simulink model "Tp7_ej5_simscape"  (R2023a)
settings: Solver=VariableStepAuto  StartTime=0.0  StopTime=2  RelTol=1e-3
libraries: fl_lib x10, nesl_utility x6, ee_lib x1, SignalEditorBlockLib x1
settings Model: Creator=Juan  LastModifiedBy=Juan

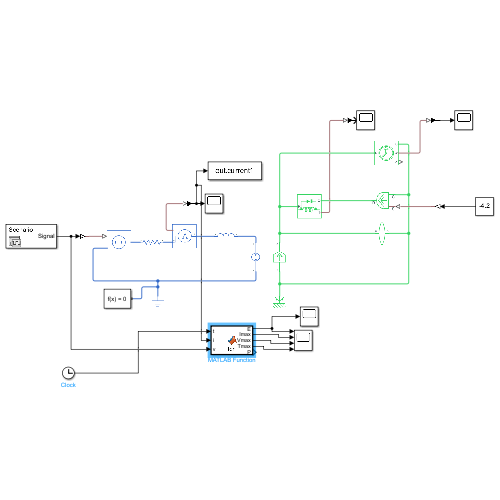
[thumbnail: Simulink's stored preview of the top-level diagram]
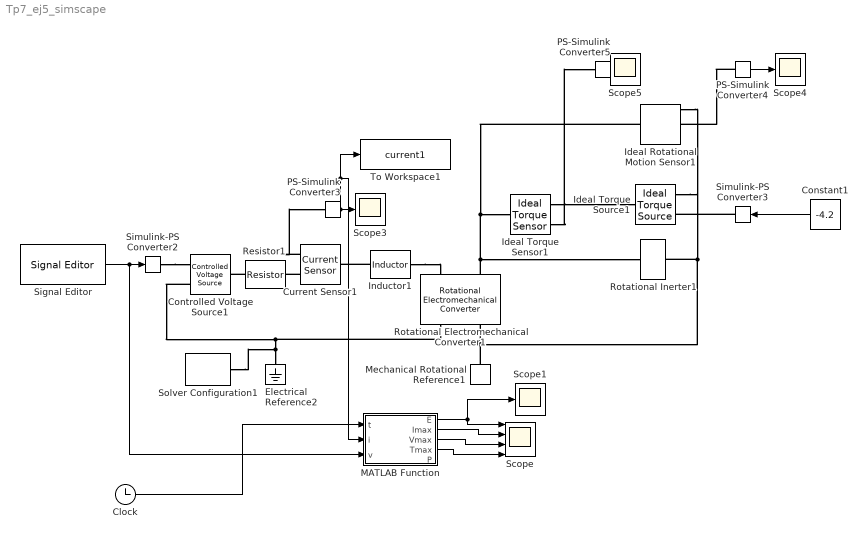
== system Tp7_ej5_simscape ==
  Clock : Clock
  Constant1 : Constant  Value=-4.2
  Controlled Voltage Source1 : fl_lib/Electrical/Electrical Sources/Controlled Voltage Source
  Current Sensor1 : fl_lib/Electrical/Electrical Sensors/Current Sensor
  Electrical Reference2 : fl_lib/Electrical/Electrical Elements/Electrical Reference
  Ideal Rotational Motion Sensor1 : fl_lib/Mechanical/Mechanical Sensors/Ideal Rotational Motion Sensor  reference=foundation.enum.MeasurementReference.difference  acceleration_port=false  velocity_port=true  position_port=true  wrap_angle=false  offset=0 rad
  Ideal Torque Sensor1 : fl_lib/Mechanical/Mechanical Sensors/Ideal Torque Sensor
  Ideal Torque Source1 : fl_lib/Mechanical/Mechanical Sources/Ideal Torque Source
  Inductor1 : ee_lib/Passive/Inductor  l=3 mH  enable_L_tol=ee.enum.toleranceApplication.none  L_tol=20  tol_distribution=ee.enum.toleranceDistribution.uniform  nSigma=4  r=0 Ohm  g=1e-9 1/Ohm  enable_operating_limits=ee.enum.enable.no  operating_limit_action=ee.enum.passive.reportOpLim.warn  max_working_current=1 A  power_rating=1 W  enable_faults=ee.enum.enable.no  fault_action=simscape.enum.assert.action.none  lambdaPercent=50  k_faulted=0.9999  turnsShort=ee.enum.passive.inductor.turnsShortOption.no  openCct=ee.enum.enable.no  groundShort=ee.enum.passive.inductor.groundShortOption.no  groundShortG=0 1/Ohm  tau_fault=1e-3 s  fault_trigger=ee.enum.faults.faultTrigger.temporal  t_fault=1 s  max_permissible_voltage=100 V  n_fail_on_voltage=1  max_permissible_current=1 A  t_fail_on_current=1 s  i_L_specify=off  i_L_priority=High  i_L=0 A  i_L_nominal_specify=off  i_L_nominal_unit=A  i_L_nominal_value=1
  MATLAB Function : MATLAB Function  TreatAsAtomicUnit=on
  Mechanical Rotational Reference1 : fl_lib/Mechanical/Rotational Elements/Mechanical Rotational Reference
  PS-Simulink Converter3 : nesl_utility/PS-Simulink Converter  PhysicalDomain=network_engine_domain  SubClassName=ps_output  LeftPortType=input  RightPortType=output  PseudoPeriodic=off  Frequencies=[]  VectorFormat=inherit  Unit=inherit  AffineConversion=off
  PS-Simulink Converter4 : nesl_utility/PS-Simulink Converter  PhysicalDomain=network_engine_domain  SubClassName=ps_output  LeftPortType=input  RightPortType=output  PseudoPeriodic=off  Frequencies=[]  VectorFormat=inherit  Unit=inherit  AffineConversion=off
  PS-Simulink Converter5 : nesl_utility/PS-Simulink Converter  PhysicalDomain=network_engine_domain  SubClassName=ps_output  LeftPortType=input  RightPortType=output  PseudoPeriodic=off  Frequencies=[]  VectorFormat=inherit  Unit=inherit  AffineConversion=off
  Resistor1 : fl_lib/Electrical/Electrical Elements/Resistor  R=4 Ohm  i_specify=off  i_priority=None  i=0 A  i_nominal_specify=off  i_nominal_unit=A  i_nominal_value=1  v_specify=off  v_priority=None  v=0 V  v_nominal_specify=off  v_nominal_unit=V  v_nominal_value=1
  Rotational Electromechanical Converter1 : fl_lib/Electrical/Electrical Elements/Rotational Electromechanical Converter  K=0.3 V*s/rad  i_specify=off  i_priority=None  i=0 A  i_nominal_specify=off  i_nominal_unit=A  i_nominal_value=1  v_specify=off  v_priority=None  v=0 V  v_nominal_specify=off  v_nominal_unit=V  v_nominal_value=1  t_specify=off  t_priority=None  t=0 N*m  t_nominal_specify=off  t_nominal_unit=N*m  t_nominal_value=1  w_specify=off  w_priority=None  w=0 rad/s  w_nominal_specify=off  w_nominal_unit=rad/s  w_nominal_value=1
  Rotational Inerter1 : fl_lib/Mechanical/Rotational Elements/Rotational Inerter  B=0.215 kg*m^2  w_specify=off  w_priority=High  w=0 rad/s  w_nominal_specify=off  w_nominal_unit=rad/s  w_nominal_value=1  t_specify=off  t_priority=None  t=0 N*m  t_nominal_specify=off  t_nominal_unit=N*m  t_nominal_value=1
      settings: InternalSimscapePortConfiguration="{\"Bottom\":[],\"Left\":[{\"id\":\"R\",\"label\":\"R\",\"type\":\"foundation.mechanical.rotational.rotational\"}],\"Right\":[{\"id\":\"C\",\"label\":\"C\",\"type\":\"foundation.mechanical.rotational.rotational\"}],\"Top\":[]}"
  Scope : Scope  NumInputPorts=4
  Scope{1,3..5} (4 alike) : Scope
  Signal Editor : SignalEditorBlockLib/Signal Editor  FileName=D:\01. Facultad\Control y Sistemas1\Control y Sistemas\Tp7\ej5.mat  ActiveScenario=Scenario  ActiveSignal=Signal  IsBus=off  OutputBusObjectStr=Bus: BusObject  SampleTime=0  Interpolate=off  ZeroCross=off  OutputAfterFinalValue=Setting to zero  Unit=inherit  PreserveSignalName=on  ApplySigPropsToAllScenarios=on
  Simulink-PS Converter2 : nesl_utility/Simulink-PS Converter  PhysicalDomain=network_engine_domain  SubClassName=ps_input  LeftPortType=input  RightPortType=output  PseudoPeriodic=off  Frequencies=[]  NoiseDistribution=none  NoiseParameters=[]  Unit=V  AffineConversion=off  FilteringAndDerivatives=provide  SimscapeFilterOrder=1  InputFilterTimeConstant=0.001  UdotUserProvided=0
  Simulink-PS Converter3 : nesl_utility/Simulink-PS Converter  PhysicalDomain=network_engine_domain  SubClassName=ps_input  LeftPortType=input  RightPortType=output  PseudoPeriodic=off  Frequencies=[]  NoiseDistribution=none  NoiseParameters=[]  Unit=N*m  AffineConversion=off  FilteringAndDerivatives=provide  SimscapeFilterOrder=1  InputFilterTimeConstant=0.001  UdotUserProvided=0
  Solver Configuration1 : nesl_utility/Solver Configuration  PhysicalDomain=network_engine_domain  SubClassName=solver  LeftPortType=input  RightPortType=generic  Tones=[]  Harmonics=[]  SimulateNoise=off  Profile=off  UseLocalSampling=off  EnableSwitchedLinearOptims=on  FrequencyDomain=off  UseCCode=off  RelTol=0.001  AbsTol=0.001  MinStep=1e-09  ToWorkspace=off  RevertToSquareIcSolve=off  NumHomotopyIterations=100  PhasorMode=off  PhasorModeNumHarmonics=1  ConsistencySolver=NEWTON_XTOL_AFTER_FTOL  IndexReductionMethod=DerivativeReplacement  DoDC=off  ResidualTolerance=1e-09  ConsistencyTolSource=GLOBAL  ConsistencyAbsTol=0.001  ConsistencyRelTol=0.001  ConsistencyTolFactor=0.001  UseLocalSolver=off  LocalSolverChoice=NE_BACKWARD_EULER_ADVANCER  ResolveIndetEquations=on  FunctionEvalNumThread=1  LocalSolverSampleTime=0.001  DoFixedCost=off  MaxNonlinIter=3  MaxModeIter=2  ComputeImpulses=off  ImpulseIterations=2  LinearAlgebra=auto  LinearAlgebraNumThread=0  EquationFormulation=NE_TIME_EF  DelaysMemoryBudget=1024  AutomaticFiltering=on  FilteringTimeConstant=0.001  PartitionStorageMethod=AS_NEEDED  PartitionMemoryBudget=1024  PartitionMethod=ROBUST
  To Workspace1 : ToWorkspace  VariableName=current1  SaveFormat=Timeseries  SampleTime=-1
  wires:
  Signal Editor/1 -> MATLAB Function/3(v), Simulink-PS Converter2/1
  PS-Simulink Converter3/1 -> MATLAB Function/2(i), To Workspace1/1, Scope3/1
  Constant1/1 -> Simulink-PS Converter3/1
  PS-Simulink Converter4/1 -> Scope4/1
  Clock/1 -> MATLAB Function/1(t)
  MATLAB Function/1(E) -> Scope/1, Scope1/1
  MATLAB Function/2(Imax) -> Scope/2
  MATLAB Function/3(Vmax) -> Scope/3
  MATLAB Function/4(Tmax) -> Scope/4
  connections:
  Controlled Voltage Source1/RConn2 -- Solver Configuration1/RConn1 -- Electrical Reference2/LConn1 -- Rotational Electromechanical Converter1/RConn1
  Simulink-PS Converter2/RConn1 -- Controlled Voltage Source1/RConn1
  Resistor1/LConn1 -- Controlled Voltage Source1/LConn1
  Inductor1/RConn1 -- Rotational Electromechanical Converter1/LConn1
  Current Sensor1/RConn2 -- Resistor1/RConn1
  Inductor1/LConn1 -- Current Sensor1/LConn1
  Current Sensor1/RConn1 -- PS-Simulink Converter3/LConn1
  Rotational Electromechanical Converter1/LConn2 -- Ideal Torque Sensor1/LConn1 -- Ideal Rotational Motion Sensor1/LConn1 -- Rotational Inerter1/LConn1
  Mechanical Rotational Reference1/LConn1 -- Rotational Electromechanical Converter1/RConn2 -- Ideal Torque Source1/RConn2 -- Ideal Rotational Motion Sensor1/RConn1 -- Rotational Inerter1/RConn1
  Simulink-PS Converter3/RConn1 -- Ideal Torque Source1/RConn1
  Ideal Torque Sensor1/RConn1 -- Ideal Torque Source1/LConn1
  PS-Simulink Converter4/LConn1 -- Ideal Rotational Motion Sensor1/RConn2
  Ideal Torque Sensor1/RConn2 -- PS-Simulink Converter5/LConn1

== matlab function Tp7_ej5_simscape/MATLAB Function ==
  settings: updateMethod=DISCRETE
  data: t input; E output; i input; v input; Imax output; Vmax output; Tmax output; P output
function [E, Imax, Vmax, Tmax, P] = fcn(t, i, v)

% t = tiempo [s]
% i = corriente [A]
% v = voltaje [V]

Kt = 0.3;   % Nm/A

persistent t_ant P_ant E_acum Imax_acum Vmax_acum Tmax_acum

if isempty(t_ant) || t <= 0

    Tm = Kt*i;

    % Potencia eléctrica consumida
    P = abs(v*i);

    E_acum = 0;
    Imax_acum = abs(i);
    Vmax_acum = abs(v);
    Tmax_acum = abs(Tm);

    t_ant = t;
    P_ant = P;
end

dt = t - t_ant;

if dt > 0

    Tm = Kt*i;

    % Uso valor absoluto para evitar problemas de signo por sensores
    P = abs(v*i);

    % Energía por regla del trapecio
    E_acum = E_acum + 0.5*(P + P_ant)*dt;

    Imax_acum = max(Imax_acum, abs(i));
    Vmax_acum = max(Vmax_acum, abs(v));
    Tmax_acum = max(Tmax_acum, abs(Tm));

    t_ant = t;
    P_ant = P;
else
    P = P_ant;
end

E    = E_acum;
Imax = Imax_acum;
Vmax = Vmax_acum;
Tmax = Tmax_acum;

end
